simulink model "Model"  (Simulink 8.5)
settings: Solver=ode8  StartTime=0.0  StopTime=0.1  FixedStep=0.1  RelTol=1e-3
values from neighbouring files (symbols this model uses):
  u1 = U1(1,i+1)    [DMC.m]    (also in VerifyingN.m; VerifyingP.m; VerifyingQ.m; VerifyingTs.m)
  u2 = U2(1,i+1)    [DMC.m]    (also in VerifyingN.m; VerifyingP.m; VerifyingQ.m; VerifyingTs.m)
  x01 = x1(end)    [DMC.m]    (also in VerifyingN.m; VerifyingP.m; VerifyingQ.m; VerifyingTs.m)
  x02 = x2(end)    [DMC.m]    (also in VerifyingN.m; VerifyingP.m; VerifyingQ.m; VerifyingTs.m)
libraries: simulink x1
settings Model: Creator=Default  LastModifiedBy=Default
settings DataIOCC: SignalLoggingSaveFormat=Dataset
settings OptimizationCC: ExpressionDepthLimit=128
settings DebuggingCC: UnderspecifiedInitializationDetection=Simplified  MergeDetectMultiDrivingBlocksExec=error  FcnCallInpInsideContextMsg=EnableAllAsError  StateNameClashWarn=none
settings GRTTargetCC: CombineOutputUpdateFcns=on  GRTInterface=off

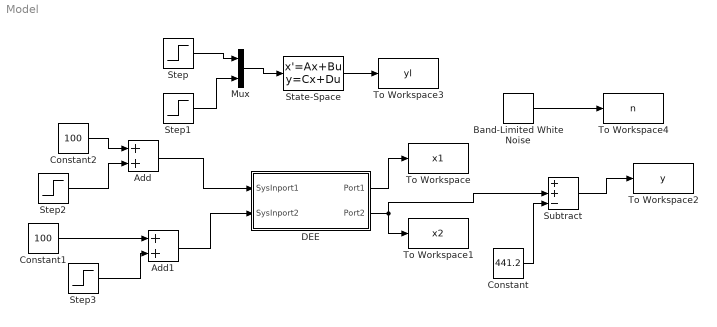
== system Model ==
  Add : Sum
  Add1 : Sum
  Band-Limited White Noise : simulink/Sources/Band-Limited White Noise  Cov=[0.01]  Ts=0.1  seed=[23341]
  Constant : Constant  Value=441.2
  Constant1 : Constant  Value=100
  Constant2 : Constant  Value=100
  DEE : Subsystem  mask(Differential Equation Editor (DEE)){}
      settings: OpenFcn=diffeqed
      mask Display: disp('Differential Equation\n Editor')
  Mux : Mux  Inputs=2
  State-Space : StateSpace  A=[-11.3 0; 2064.8 7.4]  B=[0.0091 0; -0.912 -0.9053]  C=[0 1]  D=[0 0]  X0=0
  Step : Step  Time=0  After=u1  SampleTime=0
  Step1 : Step  Time=0  After=u2  SampleTime=0
  Step2 : Step  Time=0  After=u1  SampleTime=0
  Step3 : Step  Time=0  After=u2  SampleTime=0
  Subtract : Sum  Inputs=++-
  To Workspace : ToWorkspace  VariableName=x1  SampleTime=-1
  To Workspace1 : ToWorkspace  VariableName=x2  SampleTime=-1
  To Workspace2 : ToWorkspace  VariableName=y  SampleTime=-1
  To Workspace3 : ToWorkspace  VariableName=yl  SampleTime=-1
  To Workspace4 : ToWorkspace  VariableName=n  SampleTime=-1
  wires:
  State-Space/1 -> To Workspace3/1
  Mux/1 -> State-Space/1
  Step/1 -> Mux/1
  Step1/1 -> Mux/2
  Constant1/1 -> Add1/1
  Step3/1 -> Add1/2
  Add/1 -> DEE/1(SysInport1)
  DEE/1(Port1) -> To Workspace/1
  Constant/1 -> Subtract/3
  DEE/2(Port2) -> Subtract/2, To Workspace1/1
  Subtract/1 -> To Workspace2/1
  Add1/1 -> DEE/2(SysInport2)
  Constant2/1 -> Add/1
  Step2/1 -> Add/2
  Band-Limited White Noise/1 -> To Workspace4/1

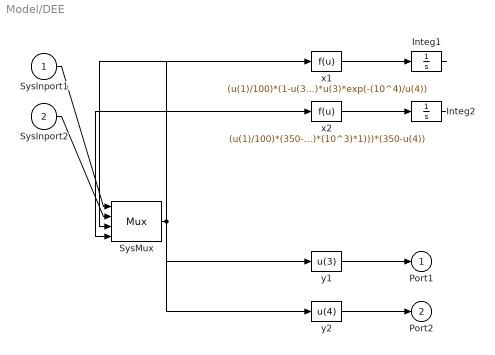
== system Model/DEE ==
  SysInport1 : Inport
  SysInport2 : Inport  Port=2
  Integ1 : Integrator  InitialCondition=x01
  Integ2 : Integrator  InitialCondition=x02
  SysMux : Mux
  x1 : Fcn  Expr=(u(1)/100)*(1-u(3))-(7.2*10^10)*u(3)*exp(-(10^4)/u(4))
  x2 : Fcn  Expr=(u(1)/100)*(350-u(4))-((-(2*10^5)/(10^3))*(7.2*10^10)*u(3)*exp(-(10^4)/u(4)))+(((10^3)*1)/((10^3)*100))*(u(2))*(1-exp(-(7*10^5)/(u(2)*(10^3)*1)))*(350-u(4))
  y1 : Fcn  Expr=u(3)
  y2 : Fcn  Expr=u(4)
  Port1 : Outport
  Port2 : Outport  Port=2
  wires:
  SysInport1/1 -> SysMux/1
  SysInport2/1 -> SysMux/2
  SysMux/1 -> x1/1, x2/1, y1/1, y2/1
  x1/1 -> Integ1/1
  Integ1/1 -> SysMux/3
  x2/1 -> Integ2/1
  Integ2/1 -> SysMux/4
  y1/1 -> Port1/1
  y2/1 -> Port2/1
